simulink model "rpendtemplatekalmann2016"  (R2016b)
settings: Solver=ode45  StartTime=0.0  StopTime=15  RelTol=1e-3  EnableMultiTasking=on
StopFcn:
  | visOutput
values from neighbouring files (symbols this model uses):
  AKC = Ad-Kk*Cd    [initLinSysID.m]
  Ce = [1 0 0 0 0 0 ... (first row only)    [initLinSysID.m]
  CTL = place(CTsys.a',CTsys.c',CTobsp)    [initLinSysID.m]
  CTsys = ss(Ae,Be,Ce,[])    [initLinSysID.m]
  DTL = place(DTsys.a',DTsys.c',DTobsp)    [initLinSysID.m]
  DTsys = c2d(CTsys,h)    [initLinSysID.m]
  Kk = Kk'    [initLinSysID.m]
undefined symbols (not defined in the file or in its folder): adingain, adinoffs, Bd, CTK, daoutgain, daoutoffs, DTK
undefined symbols (not defined in the file): h
settings Model: Creator=rbabuska  LastModifiedBy=geert
settings DataIOCC: LimitDataPoints=on  SaveFormat=Array  SignalLoggingName=sigsOut
settings OptimizationCC: BooleanDataType=off  ExpressionDepthLimit=2147483647  InitFltsAndDblsToZero=on  LifeSpan=inf
settings DebuggingCC: SaveWithParameterizedLinksMsg=none  SignalResolutionControl=TryResolveAllWithWarning  MultiTaskDSMMsg=warning  MultiTaskCondExecSysMsg=none  AllowSymbolicDim=off  StateNameClashWarn=warning  SFUnexpectedBacktrackingDiag=warning  SFNoUnconditionalDefaultTransitionDiag=warning  SFExecutionAtInitializationDiag=none
settings HardwareCC: ProdBitPerPointer=32  ProdBitPerSizeT=32  ProdBitPerPtrDiffT=32  ProdLargestAtomicFloat=None  ProdIntDivRoundTo=Undefined  ProdEndianess=Unspecified  ProdWordSize=32  ProdHWDeviceType=32-bit Generic  TargetUnknown=on
settings ModelReferenceCC: PropagateSignalLabelsOutOfModel=off
settings GRTTargetCC: TargetFcnLib=ansi_tfl_tmw.mat  TargetLangStandard=C89/C90 (ANSI)  GeneratePreprocessorConditionals=Disable all  CombineOutputUpdateFcns=off  GRTInterface=on
settings ConfigComp: CovMetricSettings=dw  CovHtmlReporting=on  CovSaveCumulativeToWorkspaceVar=on  CovSaveSingleToWorkspaceVar=on  CovExternalEMLEnable=off

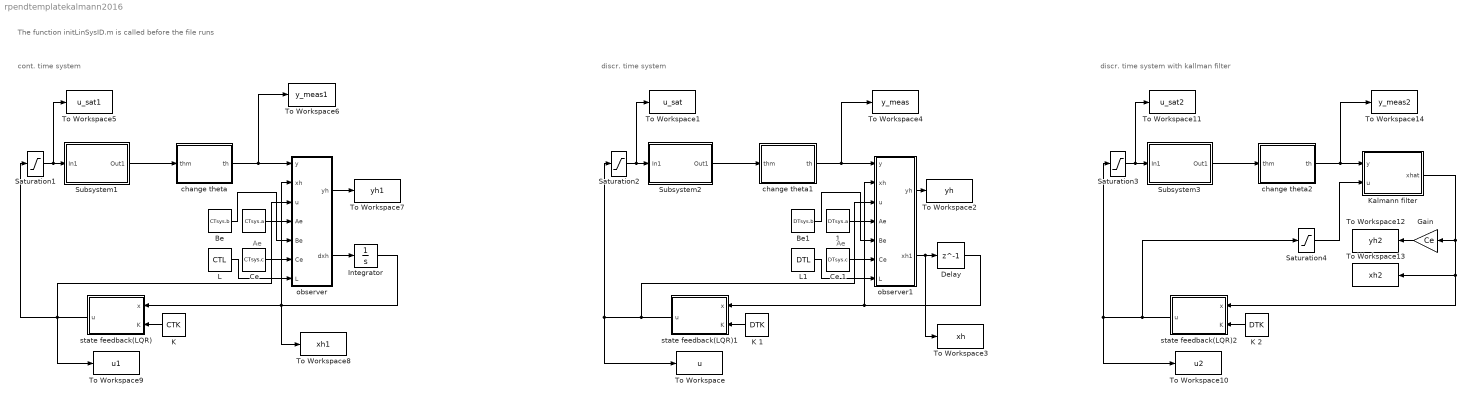
== system rpendtemplatekalmann2016 ==
  note: cont. time system
  note: Ae
  note: The function initLinSysID.m is called before the file runs
  note: discr. time system
  note: Ae
  note: discr. time system with kallman filter
  " " : Constant  Value=CTsys.a
  " 1" : Constant  Value=DTsys.a
  Be : Constant  Value=CTsys.b
  Be1 : Constant  Value=DTsys.b
  "Ce " : Constant  Value=CTsys.c
  Ce 1 : Constant  Value=DTsys.c
  Delay : Delay  DelayLength=1  InitialCondition=[0;0;0;0;0;0]
  Gain : Gain  Gain=Ce
  Integrator : Integrator  InitialCondition=[0;0;0;0;0;0]
  "K " : Constant  Value=CTK
  K 1 : Constant  Value=DTK
  K 2 : Constant  Value=DTK
  Kalmann filter : Subsystem
  L : Constant  Value=CTL
  L1 : Constant  Value=DTL
  Saturation{1..4} (4 alike) : Saturate  UpperLimit=1  LowerLimit=-1
  Subsystem1 : Subsystem
      mask Display: disp('Rotational\nPendulum')
  Subsystem2 : Subsystem
      mask Display: disp('Rotational\nPendulum')
  Subsystem3 : Subsystem
      mask Display: disp('Rotational\nPendulum')
  To Workspace : ToWorkspace  VariableName=u  SampleTime=-1
  To Workspace1 : ToWorkspace  VariableName=u_sat  SampleTime=-1
  To Workspace10 : ToWorkspace  VariableName=u2  SampleTime=-1
  To Workspace11 : ToWorkspace  VariableName=u_sat2  SampleTime=-1
  To Workspace12 : ToWorkspace  VariableName=yh2  SampleTime=-1
  To Workspace13 : ToWorkspace  VariableName=xh2  SampleTime=-1
  To Workspace14 : ToWorkspace  VariableName=y_meas2  SampleTime=-1
  To Workspace2 : ToWorkspace  VariableName=yh  SampleTime=-1
  To Workspace3 : ToWorkspace  VariableName=xh  SampleTime=-1
  To Workspace4 : ToWorkspace  VariableName=y_meas  SampleTime=-1
  To Workspace5 : ToWorkspace  VariableName=u_sat1  SampleTime=-1
  To Workspace6 : ToWorkspace  VariableName=y_meas1  SampleTime=-1
  To Workspace7 : ToWorkspace  VariableName=yh1  SampleTime=-1
  To Workspace8 : ToWorkspace  VariableName=xh1  SampleTime=-1
  To Workspace9 : ToWorkspace  VariableName=u1  SampleTime=-1
  change theta : MATLAB Function  TreatAsAtomicUnit=on
  change theta1 : MATLAB Function  TreatAsAtomicUnit=on
  change theta2 : MATLAB Function  TreatAsAtomicUnit=on
  observer : MATLAB Function  TreatAsAtomicUnit=on
  observer1 : MATLAB Function  TreatAsAtomicUnit=on
  state feedback(LQR) : MATLAB Function  TreatAsAtomicUnit=on
  state feedback(LQR)1 : MATLAB Function  TreatAsAtomicUnit=on
  state feedback(LQR)2 : MATLAB Function  TreatAsAtomicUnit=on
  wires:
  Saturation1/1 -> To Workspace5/1, Subsystem1/1(In1)
  Subsystem1/1(Out1) -> change theta/1(thm)
  change theta/1(th) -> To Workspace6/1, observer/1(y)
  observer/2(dxh) -> Integrator/1
  Integrator/1 -> To Workspace8/1, observer/2(xh), state feedback(LQR)/1(x)
  state feedback(LQR)/1(u) -> To Workspace9/1, observer/3(u), Saturation1/1
  "K "/1 -> state feedback(LQR)/2(K)
  " "/1 -> observer/4(Ae)
  Be/1 -> observer/5(Be)
  "Ce "/1 -> observer/6(Ce)
  L/1 -> observer/7(L)
  Saturation2/1 -> To Workspace1/1, Subsystem2/1(In1)
  Subsystem2/1(Out1) -> change theta1/1(thm)
  change theta1/1(th) -> To Workspace4/1, observer1/1(y)
  K 1/1 -> state feedback(LQR)1/2(K)
  " 1"/1 -> observer1/4(Ae)
  Be1/1 -> observer1/5(Be)
  Ce 1/1 -> observer1/6(Ce)
  L1/1 -> observer1/7(L)
  observer1/2(xh1) -> To Workspace3/1, Delay/1
  Delay/1 -> observer1/2(xh), state feedback(LQR)1/1(x)
  state feedback(LQR)1/1(u) -> observer1/3(u), To Workspace/1, Saturation2/1
  observer1/1(yh) -> To Workspace2/1
  observer/1(yh) -> To Workspace7/1
  state feedback(LQR)2/1(u) -> Saturation4/1, To Workspace10/1, Saturation3/1
  change theta2/1(th) -> Kalmann filter/1(y), To Workspace14/1
  K 2/1 -> state feedback(LQR)2/2(K)
  Subsystem3/1(Out1) -> change theta2/1(thm)
  Saturation3/1 -> To Workspace11/1, Subsystem3/1(In1)
  Saturation4/1 -> Kalmann filter/2(u)
  Kalmann filter/1(xhat) -> Gain/1, To Workspace13/1, state feedback(LQR)2/1(x)
  Gain/1 -> To Workspace12/1

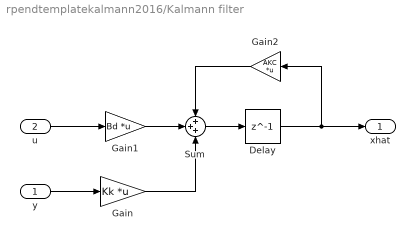
== system rpendtemplatekalmann2016/Kalmann filter ==
  y : Inport
  u : Inport  Port=2
  Delay : Delay  DelayLength=1
  Gain : Gain  Gain=Kk  Multiplication=Matrix(K*u)
  Gain1 : Gain  Gain=Bd  Multiplication=Matrix(K*u)
  Gain2 : Gain  Gain=AKC  Multiplication=Matrix(K*u)
  Sum : Sum  Inputs=+++
  xhat : Outport
  wires:
  Delay/1 -> Gain2/1, xhat/1
  y/1 -> Gain/1
  u/1 -> Gain1/1
  Sum/1 -> Delay/1
  Gain1/1 -> Sum/2
  Gain/1 -> Sum/3
  Gain2/1 -> Sum/1

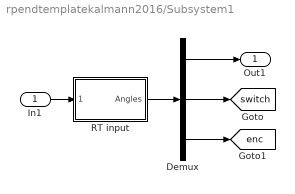
== system rpendtemplatekalmann2016/Subsystem1 ==
  In1 : Inport
  Demux : Demux  Outputs=[2 4 1]
  RT input : Subsystem  mask{Ts=h, channels=[6 7]}
      mask prompts: Ts "Sample time [s]:"; channels "Channels to read (e.g., [6 7])"
      mask init:
      | hwinit;
      | 
      | % initialize FPGA
      | fugihandle = fugiboard('Open', 'Pendulum1');
      | fugihandle.WatchdogTimeout = 0.5;
      | fugiboard('SetParams', fugihandle);
      | fugiboard('Write', fugihandle, 0, 0, 0, 0);  % dummy write to sync interface board
      | fugiboard('Write', fugihandle, 5, 1, 0, 0);  % reset position, activate relay
      | data = fugiboard('Read', fugihandle);        % get version info from FPGA
      | % model = bitshift(data(1), -5); 
      | % version = bitand(data(1), 31);
      | % disp(sprintf('FPGA setup %d, version %d', model, version)); % for the B&P it should say 1 1, or else there is a problem
      | fugiboard('Write', fugihandle, 0, 1, 0, 0);  % end reset
      | pause(0.1);                         % give relay some time to respond
      mask Display: disp('Rotational\nPendulum')
  Out1 : Outport
  tag scope: enc=global, switch=global
  wires:
  RT input/1(Angles) -> Demux/1
  Demux/1 -> Out1/1
  Demux/2 -> [switch]
  Demux/3 -> [enc]
  In1/1 -> RT input/1(Motors)

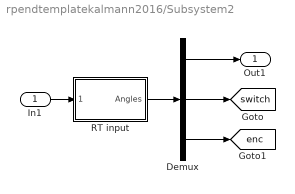
== system rpendtemplatekalmann2016/Subsystem2 ==
  In1 : Inport
  Demux : Demux  Outputs=[2 4 1]
  RT input : Subsystem  mask{Ts=h, channels=[6 7]}
      mask prompts: Ts "Sample time [s]:"; channels "Channels to read (e.g., [6 7])"
      mask init: same as rpendtemplatekalmann2016/Subsystem1/RT input
      mask Display: disp('Rotational\nPendulum')
  Out1 : Outport
  tag scope: enc=global, switch=global
  wires:
  RT input/1(Angles) -> Demux/1
  Demux/1 -> Out1/1
  Demux/2 -> [switch]
  Demux/3 -> [enc]
  In1/1 -> RT input/1(Motors)

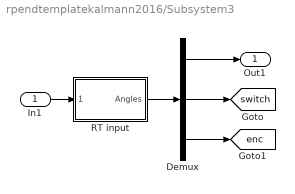
== system rpendtemplatekalmann2016/Subsystem3 ==
  In1 : Inport
  Demux : Demux  Outputs=[2 4 1]
  RT input : Subsystem  mask{Ts=h, channels=[6 7]}
      mask prompts: Ts "Sample time [s]:"; channels "Channels to read (e.g., [6 7])"
      mask init: same as rpendtemplatekalmann2016/Subsystem1/RT input
      mask Display: disp('Rotational\nPendulum')
  Out1 : Outport
  tag scope: enc=global, switch=global
  wires:
  RT input/1(Angles) -> Demux/1
  Demux/1 -> Out1/1
  Demux/2 -> [switch]
  Demux/3 -> [enc]
  In1/1 -> RT input/1(Motors)

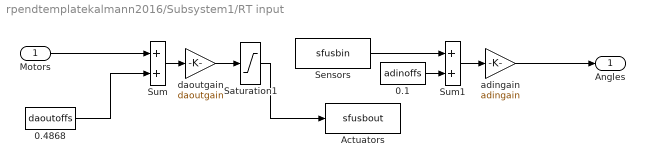
== system rpendtemplatekalmann2016/Subsystem1/RT input ==
  Motors : Inport
  0.1 : Constant  Value=adinoffs
  0.4868 : Constant  Value=daoutoffs
  Actuators : S-Function  FunctionName=sfusbout  Parameters=Ts, fugihandle  SFunctionDeploymentMode=off  EnableBusSupport=off
  Saturation1 : Saturate  UpperLimit=10  LowerLimit=-10
  Sensors : S-Function  FunctionName=sfusbin  Parameters=Ts, fugihandle, channels  SFunctionDeploymentMode=off  EnableBusSupport=off
  Sum : Sum  SaturateOnIntegerOverflow=on  InputSameDT=on  OutDataTypeStr=Inherit: Same as first input
  Sum1 : Sum  SaturateOnIntegerOverflow=on  InputSameDT=on  OutDataTypeStr=Inherit: Same as first input
  adingain : Gain  Gain=adingain  SaturateOnIntegerOverflow=on  OutDataTypeStr=Inherit: Same as input  ParamDataTypeStr=Inherit: Same as input
  daoutgain : Gain  Gain=daoutgain  SaturateOnIntegerOverflow=on  OutDataTypeStr=Inherit: Same as input  ParamDataTypeStr=Inherit: Same as input
  Angles : Outport
  wires:
  Sum/1 -> daoutgain/1
  0.4868/1 -> Sum/2
  Motors/1 -> Sum/1
  Sum1/1 -> adingain/1
  0.1/1 -> Sum1/2
  Sensors/1 -> Sum1/1
  adingain/1 -> Angles/1
  Saturation1/1 -> Actuators/1
  daoutgain/1 -> Saturation1/1

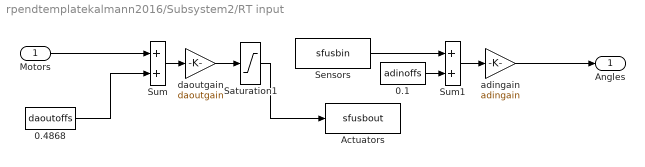
== system rpendtemplatekalmann2016/Subsystem2/RT input ==
  Motors : Inport
  0.1 : Constant  Value=adinoffs
  0.4868 : Constant  Value=daoutoffs
  Actuators : S-Function  FunctionName=sfusbout  Parameters=Ts, fugihandle  SFunctionDeploymentMode=off  EnableBusSupport=off
  Saturation1 : Saturate  UpperLimit=10  LowerLimit=-10
  Sensors : S-Function  FunctionName=sfusbin  Parameters=Ts, fugihandle, channels  SFunctionDeploymentMode=off  EnableBusSupport=off
  Sum : Sum  SaturateOnIntegerOverflow=on  InputSameDT=on  OutDataTypeStr=Inherit: Same as first input
  Sum1 : Sum  SaturateOnIntegerOverflow=on  InputSameDT=on  OutDataTypeStr=Inherit: Same as first input
  adingain : Gain  Gain=adingain  SaturateOnIntegerOverflow=on  OutDataTypeStr=Inherit: Same as input  ParamDataTypeStr=Inherit: Same as input
  daoutgain : Gain  Gain=daoutgain  SaturateOnIntegerOverflow=on  OutDataTypeStr=Inherit: Same as input  ParamDataTypeStr=Inherit: Same as input
  Angles : Outport
  wires:
  Sum/1 -> daoutgain/1
  0.4868/1 -> Sum/2
  Motors/1 -> Sum/1
  Sum1/1 -> adingain/1
  0.1/1 -> Sum1/2
  Sensors/1 -> Sum1/1
  adingain/1 -> Angles/1
  Saturation1/1 -> Actuators/1
  daoutgain/1 -> Saturation1/1

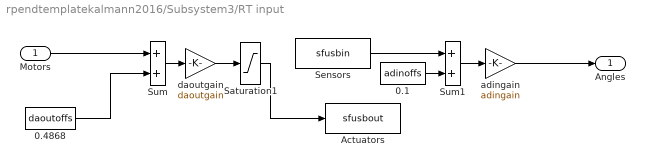
== system rpendtemplatekalmann2016/Subsystem3/RT input ==
  Motors : Inport
  0.1 : Constant  Value=adinoffs
  0.4868 : Constant  Value=daoutoffs
  Actuators : S-Function  FunctionName=sfusbout  Parameters=Ts, fugihandle  SFunctionDeploymentMode=off  EnableBusSupport=off
  Saturation1 : Saturate  UpperLimit=10  LowerLimit=-10
  Sensors : S-Function  FunctionName=sfusbin  Parameters=Ts, fugihandle, channels  SFunctionDeploymentMode=off  EnableBusSupport=off
  Sum : Sum  SaturateOnIntegerOverflow=on  InputSameDT=on  OutDataTypeStr=Inherit: Same as first input
  Sum1 : Sum  SaturateOnIntegerOverflow=on  InputSameDT=on  OutDataTypeStr=Inherit: Same as first input
  adingain : Gain  Gain=adingain  SaturateOnIntegerOverflow=on  OutDataTypeStr=Inherit: Same as input  ParamDataTypeStr=Inherit: Same as input
  daoutgain : Gain  Gain=daoutgain  SaturateOnIntegerOverflow=on  OutDataTypeStr=Inherit: Same as input  ParamDataTypeStr=Inherit: Same as input
  Angles : Outport
  wires:
  Sum/1 -> daoutgain/1
  0.4868/1 -> Sum/2
  Motors/1 -> Sum/1
  Sum1/1 -> adingain/1
  0.1/1 -> Sum1/2
  Sensors/1 -> Sum1/1
  adingain/1 -> Angles/1
  Saturation1/1 -> Actuators/1
  daoutgain/1 -> Saturation1/1

== matlab function rpendtemplatekalmann2016/state feedback(LQR) ==
  data: x input; u output; K input
function u = K(x,K)
u = -K'*x;

== matlab function rpendtemplatekalmann2016/change theta ==
  data: thm input; th output
function th = changeOfCoords(thm)
% change the measurements towards our coordinate system 
th = zeros(2,1);
th(1) = pi/2-thm(1);
th(2) = th(1)-thm(2);
% we control around up,up, thus the ref becomes
ref = [pi/2;pi/2];
th(1) = th(1)-ref(1);
th(2) = th(2)-ref(2);

== matlab function rpendtemplatekalmann2016/observer ==
  data: yh output; y input; dxh output; xh input; u input; Ae input; Be input; Ce input; L input
function [yh,dxh] = obs(y,xh,u,Ae,Be,Ce,L)
yh = Ce*xh;
dxh = Ae*xh+Be*u+L'*(y-yh);

== matlab function rpendtemplatekalmann2016/change theta1 ==
  data: thm input; th output
function th = changeOfCoords(thm)
% change the measurements towards our coordinate system 
th = zeros(2,1);
th(1) = pi/2-thm(1);
th(2) = th(1)-thm(2);
% we control around up,up, thus the ref becomes
ref = [pi/2;pi/2];
th(1) = th(1)-ref(1);
th(2) = th(2)-ref(2);

== matlab function rpendtemplatekalmann2016/observer1 ==
  data: yh output; y input; xh1 output; xh input; u input; Ae input; Be input; Ce input; L input
function [yh,xh1] = obs(y,xh,u,Ae,Be,Ce,L)
yh = Ce*xh;
xh1 = Ae*xh+Be*u+L'*(y-yh);

== matlab function rpendtemplatekalmann2016/state feedback(LQR)1 ==
  data: x input; u output; K input
function u = K(x,K)
u = -K'*x;

== matlab function rpendtemplatekalmann2016/change theta2 ==
  data: thm input; th output
function th = changeOfCoords(thm)
% change the measurements towards our coordinate system 
th = zeros(2,1);
th(1) = pi/2-thm(1);
th(2) = th(1)-thm(2);
% we control around up,up, thus the ref becomes
ref = [pi/2;pi/2];
th(1) = th(1)-ref(1);
th(2) = th(2)-ref(2);

== matlab function rpendtemplatekalmann2016/state feedback(LQR)2 ==
  data: x input; u output; K input
function u = K(x,K)
u = -K'*x;
